simulink model "Flow"  (R2022a)
settings: Solver=VariableStepAuto  StartTime=0.0  StopTime=5  RelTol=1e-3
settings Model: Creator=marks  LastModifiedBy=marks
settings DebuggingCC: AlgebraicLoopMsg=none

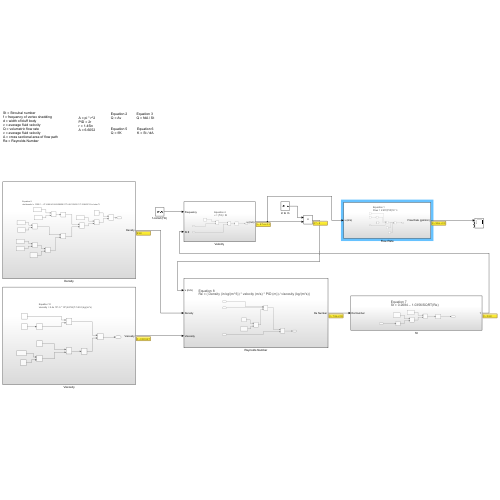
[thumbnail: Simulink's stored preview of the top-level diagram]
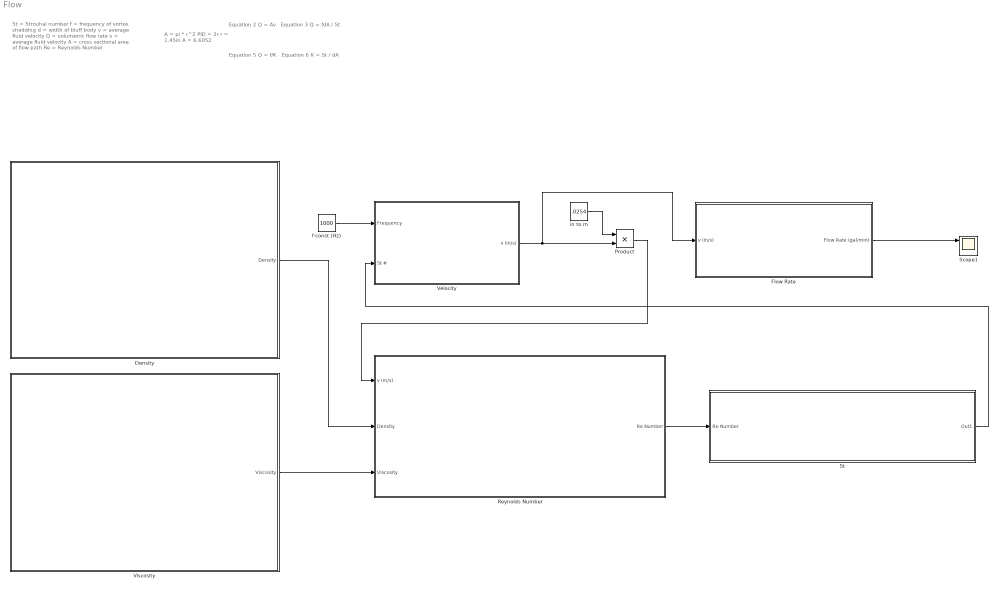
== system Flow ==
  note: A = pi * r^2
      | PID = 2r
      | r = 1.45in
      | A = 6.6052
  note: Equation 6
      | K = St / dA
  note: Equation 5
      | Q = f/K
  note: Equation 3
      | Q = fdA / St
  note: Equation 2
      | Q = Av
  note: St = Strouhal number
      | f = frequency of vortex shedding
      | d = width of bluff body
      | v = average fluid velocity
      | Q = volumetric flow rate
      | v = average fluid velocity
      | A = cross sectional area of flow path
      | Re = Reynolds Number
  Density : Subsystem
  Flow Rate : Subsystem
  Product : Product
  Reynolds Number : Subsystem
  Scope1 : Scope  NumInputPorts=3
  St : Subsystem
  Velocity : Subsystem
  Viscosity : Subsystem
  f-const (Hz) : Constant  Value=1000
  in to m : Constant  Value=.0254
  wires:
  St/1(Out1) -> Velocity/2(St #)
  Density/1(Density) -> Reynolds Number/2(Density)
  Viscosity/1(Viscosity) -> Reynolds Number/3(Viscosity)
  Reynolds Number/1(Re Number) -> St/1(Re Number)
  Flow Rate/1(Flow Rate (gal/min)) -> Scope1/1
  Product/1 -> Reynolds Number/1(v (m/s))
  in to m/1 -> Product/1
  Velocity/1(v (in/s)) -> Product/2, Flow Rate/1(v (in/s))
  f-const (Hz)/1 -> Velocity/1(Frequency)

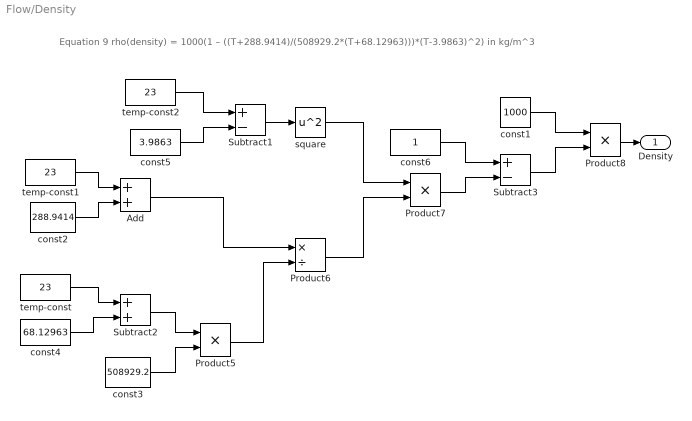
== system Flow/Density ==
  note: Equation 9
      | rho(density) = 1000(1 – ((T+288.9414)/(508929.2*(T+68.12963)))*(T-3.9863)^2) in kg/m^3
  Add : Sum  AccumDataTypeStr=double
  Product5 : Product
  Product6 : Product  Inputs=*/
  Product7 : Product
  Product8 : Product
  Subtract1 : Sum  Inputs=+-
  Subtract2 : Sum
  Subtract3 : Sum  Inputs=+-
  const1 : Constant  Value=1000
  const2 : Constant  Value=288.9414
  const3 : Constant  Value=508929.2
  const4 : Constant  Value=68.12963
  const5 : Constant  Value=3.9863
  const6 : Constant
  square : Math  Operator=square
  temp-const : Constant  Value=23
  temp-const1 : Constant  Value=23  OutDataTypeStr=double
  temp-const2 : Constant  Value=23
  Density : Outport
  wires:
  Product5/1 -> Product6/2
  Product6/1 -> Product7/2
  temp-const2/1 -> Subtract1/1
  Add/1 -> Product6/1
  const5/1 -> Subtract1/2
  const1/1 -> Product8/1
  Subtract1/1 -> square/1
  temp-const/1 -> Subtract2/1
  const3/1 -> Product5/2
  Subtract2/1 -> Product5/1
  const6/1 -> Subtract3/1
  const4/1 -> Subtract2/2
  temp-const1/1 -> Add/1
  const2/1 -> Add/2
  Subtract3/1 -> Product8/2
  Product7/1 -> Subtract3/2
  square/1 -> Product7/1
  Product8/1 -> Density/1

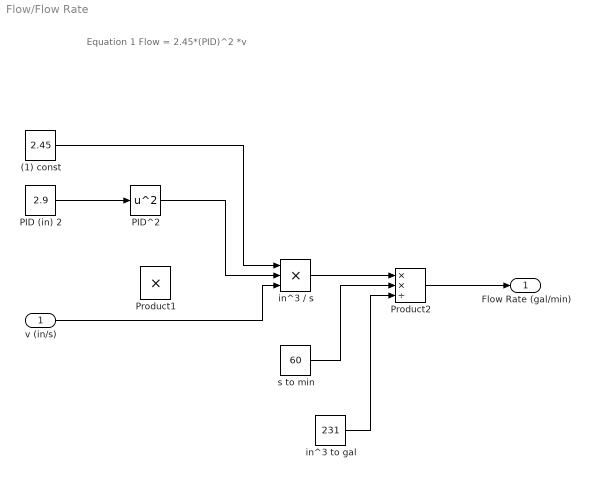
== system Flow/Flow Rate ==
  note: Equation 1
      | Flow = 2.45*(PID)^2 *v
  v (in/s) : Inport
  (1) const : Constant  Value=2.45
  PID (in) 2 : Constant  Value=2.9
  PID^2 : Math  Operator=square
  Product1 : Product
  Product2 : Product  Inputs=**/
  in^3 / s : Product  Inputs=3
  in^3 to gal : Constant  Value=231
  s to min : Constant  Value=60
  Flow Rate (gal/min) : Outport
  wires:
  PID^2/1 -> in^3 / s/2
  PID (in) 2/1 -> PID^2/1
  (1) const/1 -> in^3 / s/1
  v (in/s)/1 -> in^3 / s/3
  in^3 / s/1 -> Product2/1
  Product2/1 -> Flow Rate (gal/min)/1
  in^3 to gal/1 -> Product2/3
  s to min/1 -> Product2/2

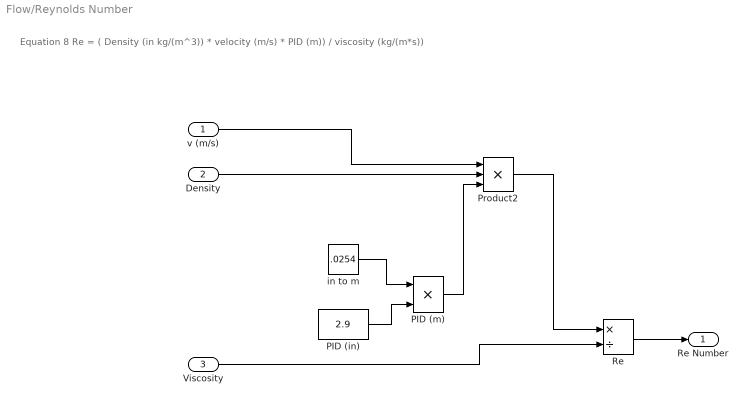
== system Flow/Reynolds Number ==
  note: Equation 8
      | Re = ( Density (in kg/(m^3)) * velocity (m/s) * PID (m)) / viscosity (kg/(m*s))
  v (m/s) : Inport
  Density : Inport  Port=2
  Viscosity : Inport  Port=3
  PID (in) : Constant  Value=2.9
  PID (m) : Product  Inputs=**
  Product2 : Product  Inputs=***
  Re : Product  Inputs=*/
  in to m : Constant  Value=.0254
  Re Number : Outport
  wires:
  Product2/1 -> Re/1
  Density/1 -> Product2/2
  v (m/s)/1 -> Product2/1
  PID (m)/1 -> Product2/3
  in to m/1 -> PID (m)/1
  PID (in)/1 -> PID (m)/2
  Viscosity/1 -> Re/2
  Re/1 -> Re Number/1

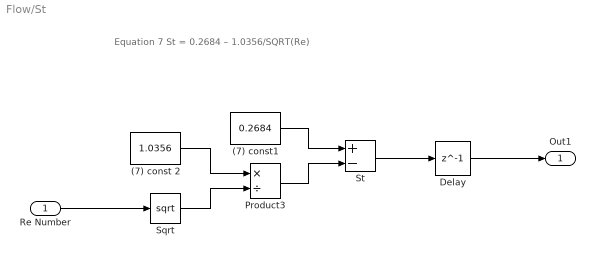
== system Flow/St ==
  note: Equation 7
      | St = 0.2684 – 1.0356/SQRT(Re)
  Re Number : Inport
  (7) const 2 : Constant  Value=1.0356
  (7) const1 : Constant  Value=0.2684
  Delay : Delay  DelayLength=1  InitialCondition=1
  Product3 : Product  Inputs=*/
  Sqrt : Sqrt
  St : Sum  Inputs=+-
  Out1 : Outport
  wires:
  (7) const 2/1 -> Product3/1
  St/1 -> Delay/1
  Product3/1 -> St/2
  Sqrt/1 -> Product3/2
  Re Number/1 -> Sqrt/1
  (7) const1/1 -> St/1
  Delay/1 -> Out1/1

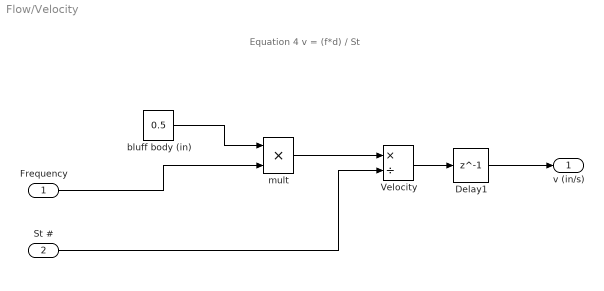
== system Flow/Velocity ==
  note: Equation 4
      | v = (f*d) / St
  Frequency : Inport
  St # : Inport  Port=2
  Delay1 : Delay  DelayLength=1  InitialCondition=1
  Velocity : Product  Inputs=*/
  bluff body (in) : Constant  Value=0.5
  mult : Product  Inputs=**
  v (in/s) : Outport
  wires:
  mult/1 -> Velocity/1
  Delay1/1 -> v (in/s)/1
  bluff body (in)/1 -> mult/1
  St #/1 -> Velocity/2
  Velocity/1 -> Delay1/1
  Frequency/1 -> mult/2

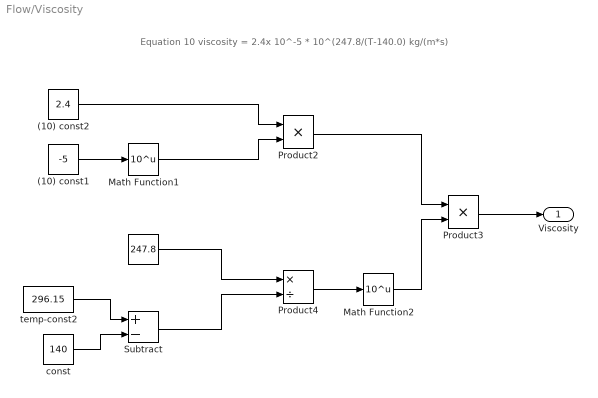
== system Flow/Viscosity ==
  note: Equation 10
      | viscosity = 2.4x 10^-5 * 10^(247.8/(T-140.0) kg/(m*s)
  " " : Constant  Value=247.8
  (10) const1 : Constant  Value=-5
  (10) const2 : Constant  Value=2.4
  Math Function1 : Math  Operator=10^u
  Math Function2 : Math  Operator=10^u
  Product2 : Product
  Product3 : Product
  Product4 : Product  Inputs=*/
  Subtract : Sum  Inputs=+-
  const : Constant  Value=140
  temp-const2 : Constant  Value=296.15
  Viscosity : Outport
  wires:
  Product2/1 -> Product3/1
  Math Function1/1 -> Product2/2
  temp-const2/1 -> Subtract/1
  Product4/1 -> Math Function2/1
  (10) const2/1 -> Product2/1
  (10) const1/1 -> Math Function1/1
  const/1 -> Subtract/2
  Math Function2/1 -> Product3/2
  Product3/1 -> Viscosity/1
  " "/1 -> Product4/1
  Subtract/1 -> Product4/2
